simulink model "Env001"  (Simulink 8.3)
settings: Solver=ode45  StartTime=0.0  StopTime=10.0  RelTol=1e-3
settings Model: Creator=swami  LastModifiedBy=swami
settings DataIOCC: SignalLoggingSaveFormat=Dataset
settings DebuggingCC: UnderspecifiedInitializationDetection=Simplified  StateNameClashWarn=none
settings GRTTargetCC: CombineOutputUpdateFcns=on  GRTInterface=off

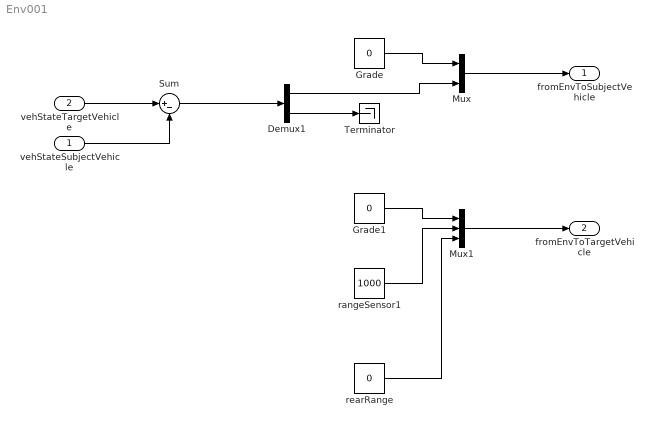
== system Env001 ==
  vehStateSubjectVehicle : Inport  PortDimensions=2
  vehStateTargetVehicle : Inport  Port=2  PortDimensions=2
  Demux1 : Demux  Outputs=2
  Grade : Constant  Value=0
  Grade1 : Constant  Value=0
  Mux : Mux  Inputs=2
  Mux1 : Mux  Inputs=3
  Sum : Sum  Inputs=|+-
  Terminator : Terminator
  rangeSensor1 : Constant  Value=1000
  rearRange : Constant  Value=0
  fromEnvToSubjectVehicle : Outport
  fromEnvToTargetVehicle : Outport  Port=2
  wires:
  vehStateSubjectVehicle/1 -> Sum/2
  Mux/1 -> fromEnvToSubjectVehicle/1
  Grade/1 -> Mux/1
  Grade1/1 -> Mux1/1
  rangeSensor1/1 -> Mux1/2
  vehStateTargetVehicle/1 -> Sum/1
  Sum/1 -> Demux1/1
  Demux1/1 -> Mux/2
  Demux1/2 -> Terminator/1
  rearRange/1 -> Mux1/3
  Mux1/1 -> fromEnvToTargetVehicle/1
